simulink model "Q2_V"  (R2023b)
settings: Solver=VariableStepAuto  StartTime=0.0  StopTime=10.0  RelTol=1e-3
settings Model: Creator=paria  LastModifiedBy=Amirali

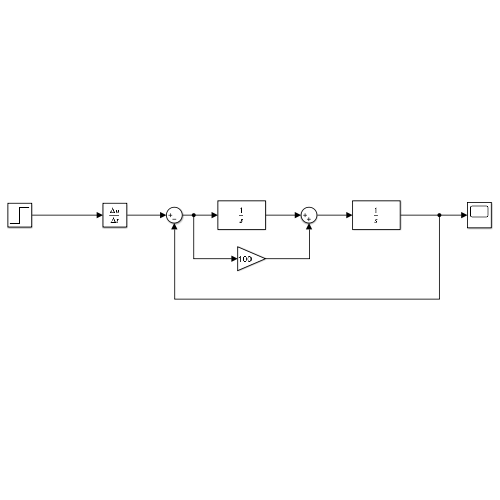
[thumbnail: Simulink's stored preview of the top-level diagram]
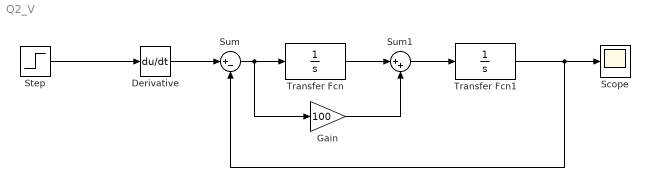
== system Q2_V ==
  Derivative : Derivative
  Gain : Gain  Gain=100
  Scope : Scope
  Step : Step  Time=0.001  SampleTime=0
  Sum : Sum  Inputs=|+-
  Sum1 : Sum  Inputs=|++
  Transfer Fcn : TransferFcn  Denominator=[1 0]
  Transfer Fcn1 : TransferFcn  Denominator=[1 0]
  wires:
  Transfer Fcn1/1 -> Sum/2, Scope/1
  Derivative/1 -> Sum/1
  Transfer Fcn/1 -> Sum1/1
  Gain/1 -> Sum1/2
  Sum/1 -> Gain/1, Transfer Fcn/1
  Step/1 -> Derivative/1
  Sum1/1 -> Transfer Fcn1/1
